simulink model "Referencegentest"  (R2023b)
settings: Solver=VariableStepAuto  StartTime=0.0  StopTime=2  RelTol=1e-3
libraries: spsCurrentMeasurementLib x7, spsSeriesRLCBranchLib x7, spsIGBTDiodeLib x4, spsVoltageMeasurementLib x4, eeGeneralControl x4, spsPLLLib x3, slpidlib x2, spsAlphaBetaZerotodq0Lib x2, spsabctoAlphaBetaZeroLib x2, spsACVoltageSourceLib x1, spsBreakerLib x1, spsDCVoltageSourceLib x1
settings Model: Creator=Jia Yee Wong  LastModifiedBy=Jia Yee Wong
settings SFSimCC: SimCustomHeaderCode="#include \"referencegen.h\""  SimUserSources=referencegen.cpp;  SimTargetLang=C++

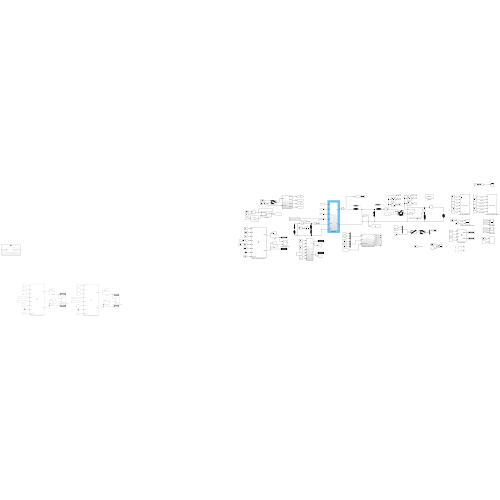
[thumbnail: Simulink's stored preview of the top-level diagram]
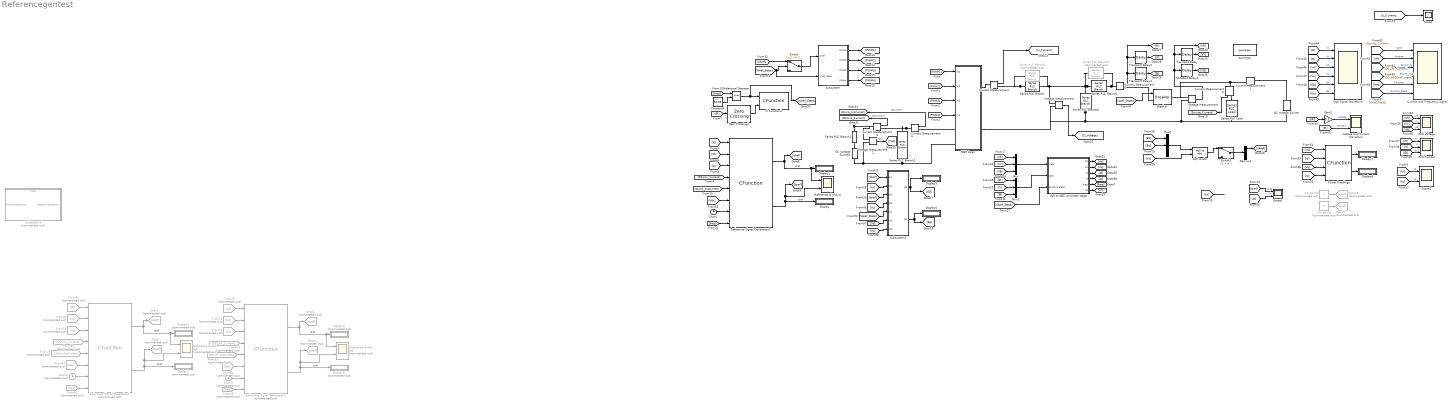
== system Referencegentest ==
  AC Voltage Source : spsACVoltageSourceLib/AC Voltage Source  Amplitude=340  Phase=0  Frequency=50  SampleTime=0  Measurements=None  BusType=PV  Pref=100  Qref=100  Qmin=-inf  Qmax=+inf
  Breaker : spsBreakerLib/Breaker  InitialState=0  SwitchingTimes="[1/60  5/60]"  External=on  BreakerResistance=0.00001  SnubberResistance=30  SnubberCapacitance=47e-9  Measurements=None  MoreParameters=on  NoBreakLoop=off
  C Function1 : CFunction  OutputCode=|  SampleTime=1/50000
      | if(Frequency == true && ZeroCross == 1){
      |     Output = 1;}
      | else if(Frequency == false){
      |         Output = 0;}
  Clock1 : Clock
  Clock2 : Clock  Commented=on
  Clock3 : Clock  Commented=on
  Constant4 : Constant  Value=50.05  SampleTime=1/50000
  Constant5 : Constant  Commented=on
  Constant6 : Constant  Commented=on  Value=0
  Current Measurement{,1..5} (6 alike) : spsCurrentMeasurementLib/Current Measurement  PhasorSimulation=off  OutputType=Complex  PSBequivalent=0
  Current and Frequency Signal : Scope  NumInputPorts=6
  DC Voltage Source1 : spsDCVoltageSourceLib/DC Voltage Source  Amplitude=400  Measurements=None
  Demux4 : Demux  Outputs=3
  Display{,1,4..7} (6 alike) : Display
  Display{2..3,8..9} (4 alike) : Display  Commented=on
  Dq0 Signal Waveform : Scope  NumInputPorts=6
  From26 : From  Commented=on  GotoTag=DCLink_OutCurrent
  From30 : From  Commented=on  GotoTag=Vdc
  From31 : From  Commented=on  GotoTag=freq
  From33 : From  Commented=on  GotoTag=DCLink_Current
  From41 : From  Commented=on  GotoTag=Id
  From42 : From  Commented=on  GotoTag=Vd
  From50 : From  Commented=on  GotoTag=Iq
  From51 : From  Commented=on  GotoTag=DCLink_OutCurrent
  From61 : From  Commented=on  GotoTag=Vdc
  From68 : From  Commented=on  GotoTag=freq
  From69 : From  Commented=on  GotoTag=DCLink_Current
  From70 : From  Commented=on  GotoTag=Id
  From71 : From  Commented=on  GotoTag=Vd
  From72 : From  Commented=on  GotoTag=Iq
  Gain2 : Gain  Gain=0.2
  Goto1 : Goto  Commented=on  GotoTag=Idref
  Goto2 : Goto  Commented=on  GotoTag=Iqref
  Goto3 : Goto  Commented=on  GotoTag=Idref
  Goto36 : Goto  Commented=on  GotoTag=Idref
  Goto37 : Goto  Commented=on  GotoTag=Iqref
  Goto4 : Goto  Commented=on  GotoTag=Iqref
  Grid Current : Scope  NumInputPorts=3
  Grid Voltage : Scope  NumInputPorts=3
  IGBT Array : Subsystem
  Mux : Mux  Inputs=3
  Mux1 : Mux  Inputs=3
  Mux2 : Mux  Inputs=3
  Power Readings : CFunction  OutputCode=|
      | PTotal = Id*Vd;
      | QTotal = Id*Vq-Vq*Id;
  Reference Id and Iq : Scope  NumInputPorts=2
  Reference Id and Iq1 : Scope  Commented=on  NumInputPorts=2
  Reference Id and Iq2 : Scope  Commented=on  NumInputPorts=2
  Reference Signal Generation1 : CFunction  Commented=on  OutputCode=|  StartCode=|  SampleTime=1/50000
      OutputCode=|
      | if(Id!=PreviousId || Iq!=PreviousIq){
      |     if(ReferenceGenTrigger(Freq_PLL)){
      |         Idref=IdrefCalc(CLK,Vd,Iin,Iout, Vdc, Vdc);
      |   //Idref =1;
      |    Iqref=0;
      |    PreviousId=Id;
      |    PreviousIq=Iq;
      |    }
      |   
      | } else { Idref = 0; Iqref = 0;}
      StartCode=|
      | PreviousIq =0;
      | PreviousId =0;
  Reference Signal Generation2 : CFunction  OutputCode=|  StartCode=|  SampleTime=1/50000
      OutputCode=|
      | if(Id!=PreviousId || Iq!=PreviousIq){
      |     if(ReferenceGenTrigger(Freq_PLL)){
      |        // Idref=IdrefCalc(CLK,Vd,Iin,Iout, Vdc, Vdc);
      |   Idref =1000/Vd;
      |    Iqref=0;
      |    PreviousId=Id;
      |    PreviousIq=Iq;
      |    }
      |   
      | } else { Idref = 0; Iqref = 0;}
      StartCode=|
      | PreviousIq =0;
      | PreviousId =0;
  Reference Signal Generation3 : CFunction  Commented=on  OutputCode=|  StartCode=|  SampleTime=1/50000
      OutputCode=|
      | if(Id!=PreviousId || Iq!=PreviousIq){
      |     if(ReferenceGenTrigger(Freq_PLL)){
      |         Idref=IdrefCalc(CLK,Vd,Iin,Iout, Vdc, Vdc);
      |   //Idref =1;
      |    Iqref=0;
      |    PreviousId=Id;
      |    PreviousIq=Iq;
      |    }
      |   
      | } else { Idref = 0; Iqref = 0;}
      StartCode=|
      | PreviousIq =0;
      | PreviousId =0;
  Relational Operator : RelationalOperator  Operator=<=  OutDataTypeStr=boolean  RndMeth=Simplest  InputSameDT=off
  Scope : Scope
  Scope1 : Scope  NumInputPorts=2
  Scope2 : Scope  NumInputPorts=2
  Series RLC Branch : spsSeriesRLCBranchLib/Series RLC Branch  LConnTagsString=__new0  RConnTagsString=__new0  BranchType=L  Resistance=1  Inductance=20.4e-3  SetiL0=off  InitialCurrent=0  Capacitance=1e-6  Setx0=off  InitialVoltage=0  Measurements=None
  Series RLC Branch1 : spsSeriesRLCBranchLib/Series RLC Branch  LConnTagsString=__new0  RConnTagsString=__new0  BranchType=L  Resistance=1  Inductance=148.336e-6  SetiL0=off  InitialCurrent=0  Capacitance=1e-6  Setx0=off  InitialVoltage=0  Measurements=None
  Series RLC Branch2 : spsSeriesRLCBranchLib/Series RLC Branch  LConnTagsString=__new0  RConnTagsString=__new0  BranchType=RC  Resistance=1  Inductance=0  SetiL0=off  InitialCurrent=0  Capacitance=47e-3  Setx0=off  InitialVoltage=300  Measurements=None
  Series RLC Branch3 : spsSeriesRLCBranchLib/Series RLC Branch  LConnTagsString=__new0  RConnTagsString=__new0  BranchType=RL  Resistance=10  Inductance=0  SetiL0=off  InitialCurrent=0  Capacitance=1e-6  Setx0=off  InitialVoltage=0  Measurements=None
  Series RLC Branch4 : spsSeriesRLCBranchLib/Series RLC Branch  Commented=on  LConnTagsString=__new0  RConnTagsString=__new0  BranchType=R  Resistance=220  Inductance=20.4e-3  SetiL0=off  InitialCurrent=0  Capacitance=1e-6  Setx0=off  InitialVoltage=0  Measurements=None
  Series RLC Branch5 : spsSeriesRLCBranchLib/Series RLC Branch  Commented=on  LConnTagsString=__new0  RConnTagsString=__new0  BranchType=R  Resistance=220  Inductance=20.4e-3  SetiL0=off  InitialCurrent=0  Capacitance=1e-6  Setx0=off  InitialVoltage=0  Measurements=None
  Series RLC Branch8 : spsSeriesRLCBranchLib/Series RLC Branch  LConnTagsString=__new0  RConnTagsString=__new0  BranchType=RC  Resistance=120  Inductance=100e-6  SetiL0=off  InitialCurrent=0  Capacitance=5.526e-6  Setx0=off  InitialVoltage=0  Measurements=None
  Series RLC Load : spsSeriesRLCLoadLib/Series RLC Load  LConnTagsString=a  RConnTagsString=__new0  NominalVoltage=240  NominalFrequency=50  ActivePower=10e2  InductivePower=0  CapacitivePower=0  Setx0=off  InitialVoltage=240  SetiL0=off  InitialCurrent=10  Measurements=None  LoadType=constant PQ
  Subsystem : Subsystem
  Subsystem3 : Subsystem
  Subsystem5 : Subsystem  Commented=on
  Switch : Switch  Threshold=1  SaturateOnIntegerOverflow=off  InputSameDT=off
  Switch5 : Switch  Threshold=1  SaturateOnIntegerOverflow=off  InputSameDT=off
  Transport Delay : TransportDelay  DelayTime=6.67e-3  BufferSize=4096
  Transport Delay1 : TransportDelay  DelayTime=13.34e-3  BufferSize=5120
  Transport Delay2 : TransportDelay  DelayTime=6.67e-3  BufferSize=4096
  Transport Delay3 : TransportDelay  DelayTime=13.34e-3  BufferSize=4096
  Voltage Measurement : spsVoltageMeasurementLib/Voltage Measurement  PhasorSimulation=off  OutputType=Complex  PSBequivalent=0
  Voltage Measurement1 : spsVoltageMeasurementLib/Voltage Measurement  PhasorSimulation=off  OutputType=Complex  PSBequivalent=0
  Voltage Measurement2 : spsVoltageMeasurementLib/Voltage Measurement  PhasorSimulation=off  OutputType=Complex  PSBequivalent=0
  Voltage and Current Waveform : Scope  NumInputPorts=2
  Zero Crossing1 : dspsigops/Zero Crossing
  dq0 to ABC converter stage : Subsystem
  dq0 to abc : spsdq0toabcLib/dq0 to abc  Alignment=90 degrees behind phase A axis
  powergui : spspowerguiLib/powergui  Priority=1  SimulationMode=Continuous  SampleTime=50e-6  frequency=60  Iterations=50  frequencyindice=0  Pbase=100e6  ErrMax=1e-4  UnitsV=kV  UnitsW=MW  buscounter=0  FunctionMessages=off  echomessages=off  EnableUseOfTLC=off  CurrentSourceSwitches=off  DisableSnubberDevices=off  DisableRonSwitches=off  DisableVfSwitches=off  DisplayEquations=off  AutomaticDiscreteSolvers=off  SolverType=Tustin/Backward Euler (TBE)  Interpol=off  ExternalGateDelay=off  methode=off  Ts=100  x0status=blocks  SPID=on  SwTol=0  HookPort=off  NonlinearTolerance=1e-4  nMaxIteration=100  ContinueOnMaxIteration=off  RestoreLinks=warning  ResistiveCurrentMeasurement=off  Frange=[0:2:500]  Ylog=off  Xlog=on  ShowGrid=off  save=off  variable=ZData  structure=0  ZoomFFT=off  StartTime=0.0  cycles=1  DisplayStyle=1  fundamental=60  FreqAxis=off  MaxFrequency=1000  frequencyindicesteady=1  RmsSteady=1  display=off
  wires:
  [IR] -> Voltage and Current Waveform/2  "Current"
  Clock1/1 -> Reference Signal Generation2/7
  [Vq] -> Subsystem3/7(In6)
  [Iq] -> Power Readings/4
  Subsystem/4(PWM4) -> [PWM4]
  [VAref_State] -> dq0 to ABC converter stage/3(Synchro State)
  [VAref_State] -> Subsystem3/5(In2)
  Switch/1 -> Subsystem/1(Vref)
  Constant5/1 -> Goto36/1
  [Iq] -> Subsystem3/4(In8)
  [Vdc] -> Reference Signal Generation2/6
  [Id] -> Power Readings/2
  [DCLink_Current] -> Reference Signal Generation2/4
  Reference Signal Generation2/2 -> Reference Id and Iq/2, [Iqref], Display/1  "Iqref"
  [IR] -> Mux1/1
  dq0 to ABC converter stage/2(Vq) -> [Vq]
  [Iq] -> Reference Signal Generation2/3
  [Id] -> Subsystem3/2(In4)
  Current Measurement3/1 -> [DCLink_Current]  "DCLinkOut"
  Transport Delay3/1 -> [IB]
  dq0 to ABC converter stage/4(Iq) -> [Iq]
  Switch5/1 -> Demux4/1
  Mux/1 -> dq0 to ABC converter stage/1(Vabc)
  Subsystem3/1(Ed) -> [ED], Display5/1
  [VY] -> Grid Voltage/2  "VY"
  [VR] -> Mux/1
  [IY] -> Grid Current/2  "IY"
  dq0 to abc/1 -> Switch5/1
  Subsystem/1(PWM1) -> [PWM1]
  [VR] -> Grid Voltage/1  "VR"
  [wt] -> dq0 to abc/2
  [VAref] -> Switch/1
  [freq] -> Relational Operator/1
  Constant4/1 -> Relational Operator/2
  [VB] -> Grid Voltage/3  "VB"
  Subsystem/2(PWM2) -> [PWM2]
  Current Measurement/1 -> [Li_Current]
  Transport Delay1/1 -> [VB]
  Transport Delay2/1 -> [IY]
  Transport Delay/1 -> [VY]
  Mux2/1 -> dq0 to abc/1
  dq0 to ABC converter stage/3(Id) -> [Id]
  [VAref_State] -> Breaker/1
  [VR] -> Gain2/1
  Relational Operator/1 -> [VAref_State], C Function1/1
  [freq] -> Reference Signal Generation2/8
  dq0 to ABC converter stage/5(freq) -> [freq]
  [Eq] -> Mux2/2
  [IR] -> Current and Frequency Signal/2  "Iinverter"
  [Id] -> Scope2/1  "Id"
  Constant6/1 -> Goto37/1
  [Vd] -> Dq0 Signal Waveform/3  "Vd"
  Zero Crossing1/1 -> C Function1/2
  Current Measurement4/1 -> [DCLink_OutCurrent]  "DCLinkIN"
  [IR] -> Zero Crossing1/1
  [Source_Current] -> Current and Frequency Signal/1  "Igrid"
  [VAref_State] -> Current and Frequency Signal/6  "Synchro_State"
  Voltage Measurement2/1 -> [Vdc]  "VDC"
  [Iqref] -> Subsystem3/3(In5)
  Current Measurement1/1 -> [IR], Transport Delay2/1, Transport Delay3/1
  Gain2/1 -> Voltage and Current Waveform/1  "Voltage"
  [Vq] -> Dq0 Signal Waveform/4  "Vq"
  Subsystem/3(PWM3) -> [PWM3]
  [IB] -> Grid Current/3  "IB"
  [Vd] -> Reference Signal Generation2/2
  [DCLink_OutCurrent] -> Current and Frequency Signal/4  "DCLink_Out"
  [Id] -> Reference Signal Generation2/1
  [PWM2] -> IGBT Array/2(In1)
  [DCLink_Current] -> Current and Frequency Signal/3  "DcLink_IN"
  dq0 to ABC converter stage/1(Vd) -> [Vd]
  [ED] -> Mux2/1
  [PWM3] -> IGBT Array/3(In3)
  [ED] -> Dq0 Signal Waveform/5  "Ed"
  Voltage Measurement1/1 -> [VR], Transport Delay/1, Transport Delay1/1
  [IY] -> Mux1/2
  [Idref] -> Subsystem3/1(In1)
  [VY] -> Mux/2
  Power Readings/1 -> Display7/1
  [IR] -> Grid Current/1  "IR"
  [Vq] -> Power Readings/3
  [PWM1] -> IGBT Array/1(In2)
  [IB] -> Mux1/3
  [VB] -> Mux/3
  [Vd] -> Power Readings/1
  Power Readings/2 -> Display4/1
  Reference Signal Generation2/1 -> Reference Id and Iq/1, Display1/1, [Idref]  "Idref"
  [PWM4] -> IGBT Array/4(In4)
  Demux4/1 -> [VAref]
  Voltage Measurement/1 -> [Ci_Voltage]
  Current Measurement5/1 -> [Source_Current]
  Subsystem3/2(Eq) -> [Eq], Display6/1
  dq0 to ABC converter stage/6(wt) -> [wt]
  [DCLink_OutCurrent] -> Reference Signal Generation2/5
  [freq] -> Current and Frequency Signal/5  "FSystem"
  Mux1/1 -> dq0 to ABC converter stage/2(IAbc)
  [Id] -> Dq0 Signal Waveform/1  "Id"
  [Iq] -> Dq0 Signal Waveform/2  "Iq"
  [Eq] -> Dq0 Signal Waveform/6  "Eq"
  [Iq] -> Scope2/2  "Iq"
  [Vd] -> Subsystem3/6(In3)
  [VAref_State] -> Subsystem/2(Vref_state), Switch/2
  Reference Signal Generation1/1 -> Reference Id and Iq1/1, Display3/1, Goto1/1  "Idref"
  From26/1 -> Reference Signal Generation1/5
  From42/1 -> Reference Signal Generation1/2
  From50/1 -> Reference Signal Generation1/3
  From31/1 -> Reference Signal Generation1/8
  Reference Signal Generation1/2 -> Reference Id and Iq1/2, Goto2/1, Display2/1  "Iqref"
  Clock2/1 -> Reference Signal Generation1/7
  From30/1 -> Reference Signal Generation1/6
  From33/1 -> Reference Signal Generation1/4
  From41/1 -> Reference Signal Generation1/1
  From70/1 -> Reference Signal Generation3/1
  Clock3/1 -> Reference Signal Generation3/7
  From69/1 -> Reference Signal Generation3/4
  Reference Signal Generation3/2 -> Reference Id and Iq2/2, Goto4/1, Display8/1  "Iqref"
  From68/1 -> Reference Signal Generation3/8
  From61/1 -> Reference Signal Generation3/6
  From72/1 -> Reference Signal Generation3/3
  From71/1 -> Reference Signal Generation3/2
  From51/1 -> Reference Signal Generation3/5
  Reference Signal Generation3/1 -> Reference Id and Iq2/1, Display9/1, Goto3/1  "Idref"
  [Id] -> Scope1/2  "Id"
  [Idref] -> Scope1/1  "Idref"
  [Li_Current] -> Scope/1
  [wt] -> ?
  connections:
  Current Measurement4/LConn1 -- Current Measurement3/RConn1 -- Series RLC Branch2/LConn1
  Series RLC Branch8/RConn1 -- IGBT Array/RConn2 -- Voltage Measurement/LConn2 -- AC Voltage Source/LConn1 -- Series RLC Load/RConn1 -- Voltage Measurement1/LConn2
  Voltage Measurement2/LConn2 -- Series RLC Branch2/RConn1 -- IGBT Array/LConn2 -- DC Voltage Source1/LConn1
  Series RLC Branch1/LConn1 -- Series RLC Branch8/LConn1 -- Series RLC Branch5/LConn1 -- Voltage Measurement/LConn1 -- Series RLC Branch/RConn1 -- Series RLC Branch4/RConn1
  Series RLC Branch3/LConn1 -- Current Measurement3/LConn1 -- Voltage Measurement2/LConn1
  Current Measurement1/LConn1 -- Series RLC Branch5/RConn1 -- Series RLC Branch1/RConn1
  Current Measurement2/RConn1 -- Breaker/RConn1 -- Voltage Measurement1/LConn1 -- Current Measurement5/LConn1
  Series RLC Branch/LConn1 -- Current Measurement/RConn1 -- Series RLC Branch4/LConn1
  IGBT Array/RConn1 -- Current Measurement/LConn1
  Current Measurement4/RConn1 -- IGBT Array/LConn1
  Breaker/LConn1 -- Current Measurement1/RConn1
  Current Measurement2/LConn1 -- AC Voltage Source/RConn1
  Current Measurement5/RConn1 -- Series RLC Load/LConn1
  Series RLC Branch3/RConn1 -- DC Voltage Source1/RConn1

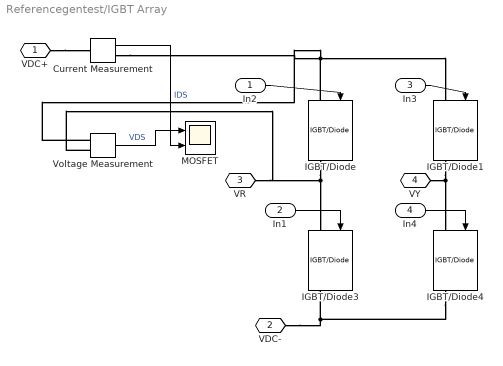
== system Referencegentest/IGBT Array ==
  In2 : Inport
  In1 : Inport  Port=2
  In3 : Inport  Port=3
  In4 : Inport  Port=4
  Current Measurement : spsCurrentMeasurementLib/Current Measurement  PhasorSimulation=off  OutputType=Complex  PSBequivalent=0
  IGBT/Diode{,1,3..4} (4 alike) : spsIGBTDiodeLib/IGBT//Diode  Ron=1e-3  Rs=1e5  Cs=inf  Measurements=on
  MOSFET : Scope  NumInputPorts=2
  Voltage Measurement : spsVoltageMeasurementLib/Voltage Measurement  PhasorSimulation=off  OutputType=Complex  PSBequivalent=0
  VDC+ : PMIOPort  Side=Left
  VDC- : PMIOPort  Port=2  Side=Left
  VR : PMIOPort  Port=3  Side=Right
  VY : PMIOPort  Port=4  Side=Right
  wires:
  In1/1 -> IGBT/Diode3/1
  In4/1 -> IGBT/Diode4/1
  In3/1 -> IGBT/Diode1/1
  In2/1 -> IGBT/Diode/1
  Voltage Measurement/1 -> MOSFET/1  "VDS"
  Current Measurement/1 -> MOSFET/2  "IDS"
  connections:
  IGBT/Diode4/RConn1 -- VDC-/RConn1 -- IGBT/Diode3/RConn1
  IGBT/Diode/RConn1 -- Voltage Measurement/LConn2 -- VR/RConn1 -- IGBT/Diode3/LConn1
  IGBT/Diode1/RConn1 -- VY/RConn1 -- IGBT/Diode4/LConn1
  IGBT/Diode/LConn1 -- Current Measurement/RConn1 -- Voltage Measurement/LConn1 -- IGBT/Diode1/LConn1
  VDC+/RConn1 -- Current Measurement/LConn1

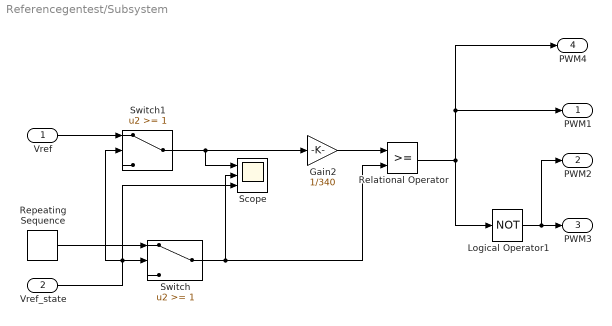
== system Referencegentest/Subsystem ==
  Vref : Inport
  Vref_state : Inport  Port=2
  Gain2 : Gain  Gain=1/340
  Logical Operator1 : Logic  Operator=NOT  AllPortsSameDT=off  OutDataTypeStr=boolean
  Relational Operator : RelationalOperator  OutDataTypeStr=boolean  RndMeth=Simplest  InputSameDT=off
  Repeating Sequence : simulink/Sources/Repeating Sequence  rep_seq_t=[0 0.00005 0.0001]  rep_seq_y=[-1 1 -1]
  Scope : Scope  NumInputPorts=3
  Switch : Switch  Threshold=1  SaturateOnIntegerOverflow=off  InputSameDT=off
  Switch1 : Switch  Threshold=1  SaturateOnIntegerOverflow=off  InputSameDT=off
  PWM1 : Outport
  PWM2 : Outport  Port=2
  PWM3 : Outport  Port=3
  PWM4 : Outport  Port=4
  wires:
  Gain2/1 -> Relational Operator/1
  Relational Operator/1 -> Logical Operator1/1, PWM1/1, PWM4/1
  Logical Operator1/1 -> PWM2/1, PWM3/1
  Repeating Sequence/1 -> Switch/1
  Switch/1 -> Scope/2, Relational Operator/2
  Vref_state/1 -> Scope/3, Switch1/2, Switch/2
  Switch1/1 -> Gain2/1, Scope/1
  Vref/1 -> Switch1/1

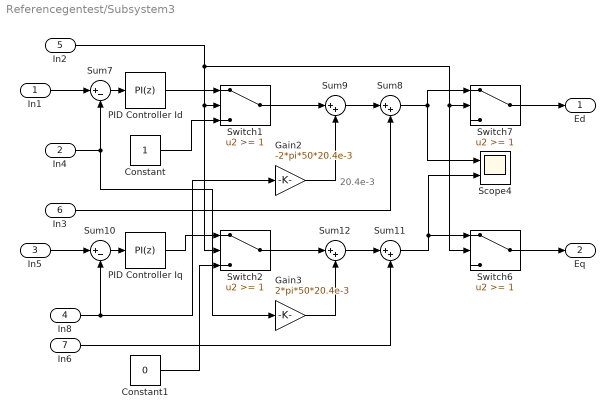
== system Referencegentest/Subsystem3 ==
  note: 20.4e-3
  In1 : Inport
  In4 : Inport  Port=2
  In5 : Inport  Port=3
  In8 : Inport  Port=4
  In2 : Inport  Port=5
  In3 : Inport  Port=6
  In6 : Inport  Port=7
  Constant : Constant
  Constant1 : Constant  Value=0
  Gain2 : Gain  Gain=-2*pi*50*20.4e-3
  Gain3 : Gain  Gain=2*pi*50*20.4e-3
  PID Controller Id : slpidlib/PID Controller  Controller=PI  Form=Parallel  TimeDomain=Discrete-time  UseExternalTs=off  SampleTime=5e-5  IntegratorMethod=Forward Euler  FilterMethod=Forward Euler  ControllerParametersSource=internal  P=500  I=100  UseKiTs=on  D=0.2  N=100  UseFilter=on  TunerSelectOption=Transfer Function Based (PID Tuner App)  InitialConditionSource=internal  InitialConditionForIntegrator=0  InitialConditionForFilter=0  DifferentiatorICPrevScaledInput=0  ExternalReset=none  TrackingMode=off  Kt=1  LimitOutput=on  SatLimitsSource=internal  UpperSaturationLimit=200  LowerSaturationLimit=-200  LinearizeAsGain=on  AntiWindupMode=back-calculation  Kb=1  LimitIntegrator=off  UpperIntegratorSaturationLimit=inf  LowerIntegratorSaturationLimit=-inf  POutMin=[]  POutMax=[]  IOutMin=[]  IOutMax=[]  DOutMin=[]  DOutMax=[]  NOutMin=[]  NOutMax=[]  SumOutMin=[]  SumOutMax=[]  SaturationOutMin=[]  SaturationOutMax=[]  PParamMin=[]  PParamMax=[]  IParamMin=[]  IParamMax=[]  DParamMin=[]  DParamMax=[]  NParamMin=[]  NParamMax=[]  KbParamMin=[]  KbParamMax=[]  KtParamMin=[]  KtParamMax=[]  KbOutMin=[]  KbOutMax=[]  KtOutMin=[]  KtOutMax=[]  IntegratorOutMin=[]  IntegratorOutMax=[]  FilterOutMin=[]  FilterOutMax=[]  SumI1OutMin=[]  SumI1OutMax=[]  SumI2OutMin=[]  SumI2OutMax=[]  SumI3OutMin=[]  SumI3OutMax=[]  SumI4OutMin=[]  SumI4OutMax=[]  SumDOutMin=[]  SumDOutMax=[]  DifferentiatorOutMin=[]  DifferentiatorOutMax=[]  FilterDiffOutCoefMin=[]  FilterDiffOutCoefMax=[]  ReciprocalOutMin=[]  ReciprocalOutMax=[]  SumDenOutMin=[]  SumDenOutMax=[]  SumNumOutMin=[]  SumNumOutMax=[]  DivideOutMin=[]  DivideOutMax=[]  UdiffTsProdOutMin=[]  UdiffTsProdOutMax=[]  NTsProdOutMin=[]  NTsProdOutMax=[]  UintegralTsProdOutMin=[]  UintegralTsProdOutMax=[]  UngainTsProdOutMin=[]  UngainTsProdOutMax=[]  ClampingZeroOutDataTypeStr=Inherit: Inherit via back propagation  ClampingZeroOutMin=[]  ClampingZeroOutMax=[]  FilterDenConstantOutDataTypeStr=Inherit: Inherit via back propagation  FilterDenConstantOutMin=[]  FilterDenConstantOutMax=[]  PCopyOutDataTypeStr=Inherit: Inherit via back propagation  PCopyOutMin=[]  PCopyOutMax=[]  NCopyOutDataTypeStr=Inherit: Inherit via back propagation  NCopyOutMin=[]  NCopyOutMax=[]  IntegratorContinuousStateAttributes=''  IntegratorStateIdentifier=Id  IntegratorStateMustResolveToSignalObject=off  IntegratorRTWStateStorageClass=Auto  FilterContinuousStateAttributes=''  FilterStateMustResolveToSignalObject=off  FilterRTWStateStorageClass=Auto  ParallelPVariant=InternalParameters  IdealPVariant=Disabled  IVariant=InternalParameters  DVariant=Disabled  IntegratorVariant=Discrete  SatVariant=Enabled  AWVariant=BackCalculation  PCopyVariant=Disabled  TRVariant=Disabled  FdbkBlocksVariant=Forward  IdealPFdbkVariant=Disabled  SatFdbkVariant=Disabled  DerivativeFilterVariant=Disabled  NVariant=Disabled  NCopyVariant=Disabled_SignalSpec  FilterICVariant=Disabled  IntegratorICVariant=InternalICs  ExternalResetVariant=Disabled  TRSumVariant=Passthrough  SumFdbkVariant=Disabled  SumVariant=Sum_PI  TsampFilterVariant=InternalTs  TsampNgainVariant=Passthrough  TsampIntegralVariant=Disabled_SignalSpec  ExternalSaturationOutDataTypeStr=Inherit: Same as second input
  PID Controller Iq : slpidlib/PID Controller  Controller=PI  Form=Parallel  TimeDomain=Discrete-time  UseExternalTs=off  SampleTime=5e-5  IntegratorMethod=Forward Euler  FilterMethod=Forward Euler  ControllerParametersSource=internal  P=500  I=100  UseKiTs=on  D=0.2  N=100  UseFilter=on  TunerSelectOption=Transfer Function Based (PID Tuner App)  InitialConditionSource=internal  InitialConditionForIntegrator=0  InitialConditionForFilter=0  DifferentiatorICPrevScaledInput=0  ExternalReset=none  TrackingMode=off  Kt=1  LimitOutput=on  SatLimitsSource=internal  UpperSaturationLimit=200  LowerSaturationLimit=-200  LinearizeAsGain=on  AntiWindupMode=back-calculation  Kb=1  LimitIntegrator=off  UpperIntegratorSaturationLimit=inf  LowerIntegratorSaturationLimit=-inf  POutMin=[]  POutMax=[]  IOutMin=[]  IOutMax=[]  DOutMin=[]  DOutMax=[]  NOutMin=[]  NOutMax=[]  SumOutMin=[]  SumOutMax=[]  SaturationOutMin=[]  SaturationOutMax=[]  PParamMin=[]  PParamMax=[]  IParamMin=[]  IParamMax=[]  DParamMin=[]  DParamMax=[]  NParamMin=[]  NParamMax=[]  KbParamMin=[]  KbParamMax=[]  KtParamMin=[]  KtParamMax=[]  KbOutMin=[]  KbOutMax=[]  KtOutMin=[]  KtOutMax=[]  IntegratorOutMin=[]  IntegratorOutMax=[]  FilterOutMin=[]  FilterOutMax=[]  SumI1OutMin=[]  SumI1OutMax=[]  SumI2OutMin=[]  SumI2OutMax=[]  SumI3OutMin=[]  SumI3OutMax=[]  SumI4OutMin=[]  SumI4OutMax=[]  SumDOutMin=[]  SumDOutMax=[]  DifferentiatorOutMin=[]  DifferentiatorOutMax=[]  FilterDiffOutCoefMin=[]  FilterDiffOutCoefMax=[]  ReciprocalOutMin=[]  ReciprocalOutMax=[]  SumDenOutMin=[]  SumDenOutMax=[]  SumNumOutMin=[]  SumNumOutMax=[]  DivideOutMin=[]  DivideOutMax=[]  UdiffTsProdOutMin=[]  UdiffTsProdOutMax=[]  NTsProdOutMin=[]  NTsProdOutMax=[]  UintegralTsProdOutMin=[]  UintegralTsProdOutMax=[]  UngainTsProdOutMin=[]  UngainTsProdOutMax=[]  ClampingZeroOutDataTypeStr=Inherit: Inherit via back propagation  ClampingZeroOutMin=[]  ClampingZeroOutMax=[]  FilterDenConstantOutDataTypeStr=Inherit: Inherit via back propagation  FilterDenConstantOutMin=[]  FilterDenConstantOutMax=[]  PCopyOutDataTypeStr=Inherit: Inherit via back propagation  PCopyOutMin=[]  PCopyOutMax=[]  NCopyOutDataTypeStr=Inherit: Inherit via back propagation  NCopyOutMin=[]  NCopyOutMax=[]  IntegratorContinuousStateAttributes=''  IntegratorStateIdentifier=Id  IntegratorStateMustResolveToSignalObject=off  IntegratorRTWStateStorageClass=Auto  FilterContinuousStateAttributes=''  FilterStateMustResolveToSignalObject=off  FilterRTWStateStorageClass=Auto  ParallelPVariant=InternalParameters  IdealPVariant=Disabled  IVariant=InternalParameters  DVariant=Disabled  IntegratorVariant=Discrete  SatVariant=Enabled  AWVariant=BackCalculation  PCopyVariant=Disabled  TRVariant=Disabled  FdbkBlocksVariant=Forward  IdealPFdbkVariant=Disabled  SatFdbkVariant=Disabled  DerivativeFilterVariant=Disabled  NVariant=Disabled  NCopyVariant=Disabled_SignalSpec  FilterICVariant=Disabled  IntegratorICVariant=InternalICs  ExternalResetVariant=Disabled  TRSumVariant=Passthrough  SumFdbkVariant=Disabled  SumVariant=Sum_PI  TsampFilterVariant=InternalTs  TsampNgainVariant=Passthrough  TsampIntegralVariant=Disabled_SignalSpec  ExternalSaturationOutDataTypeStr=Inherit: Same as second input
  Scope4 : Scope  NumInputPorts=2
  Sum10 : Sum  Inputs=|+-
  Sum{8..9,11..12} (4 alike) : Sum  Inputs=|++
  Sum7 : Sum  Inputs=|+-
  Switch{1..2,6..7} (4 alike) : Switch  Threshold=1  SaturateOnIntegerOverflow=off  InputSameDT=off
  Ed : Outport
  Eq : Outport  Port=2
  wires:
  Switch1/1 -> Sum9/1
  In5/1 -> Sum10/1
  In1/1 -> Sum7/1
  In6/1 -> Sum11/2
  In2/1 -> Switch6/2, Switch7/2, Switch2/2, Switch1/2
  Switch7/1 -> Ed/1
  Sum8/1 -> Scope4/1, Switch7/1
  Sum10/1 -> PID Controller Iq/1
  Sum11/1 -> Switch6/1, Scope4/2
  Gain3/1 -> Sum12/2
  Sum7/1 -> PID Controller Id/1
  PID Controller Iq/1 -> Switch2/1
  In3/1 -> Sum8/2
  Sum9/1 -> Sum8/1
  Gain2/1 -> Sum9/2
  Sum12/1 -> Sum11/1
  In4/1 -> Gain3/1, Sum7/2
  In8/1 -> Gain2/1, Sum10/2
  PID Controller Id/1 -> Switch1/1
  Switch2/1 -> Sum12/1
  Switch6/1 -> Eq/1
  Constant/1 -> Switch1/3
  Constant1/1 -> Switch2/3

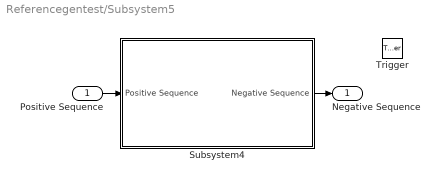
== system Referencegentest/Subsystem5 ==
  Positive Sequence : Inport
  Trigger : TriggerPort  VariantControl=(inherit)  PortDimensions=1
  Subsystem4 : Subsystem
  Negative Sequence : Outport
  wires:
  Subsystem4/1(Negative Sequence) -> Negative Sequence/1
  Positive Sequence/1 -> Subsystem4/1(Positive Sequence)

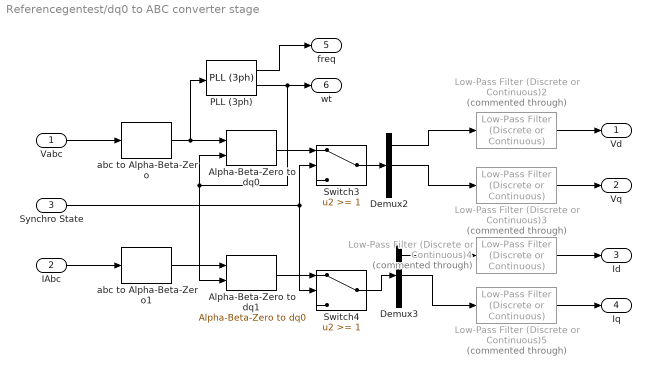
== system Referencegentest/dq0 to ABC converter stage ==
  Vabc : Inport
  IAbc : Inport  Port=2
  Synchro State : Inport  Port=3
  Alpha-Beta-Zero to dq0 : spsAlphaBetaZerotodq0Lib/Alpha-Beta-Zero to dq0  Alignment=90 degrees behind phase A axis
  Alpha-Beta-Zero to dq1 : spsAlphaBetaZerotodq0Lib/Alpha-Beta-Zero to dq0  Alignment=90 degrees behind phase A axis
  Demux2 : Demux  Outputs=3
  Demux3 : Demux  Outputs=3
  Low-Pass Filter (Discrete or Continuous){2..5} (4 alike) : eeGeneralControl/Low-Pass Filter (Discrete or Continuous)  Commented=through  K=1  T=2*pi*50  B=inf  A=-inf  init_option=Inherited from block input  x0=0  Ts=0
  PLL (3ph) : spsPLL3phLib/PLL (3ph)  Fmin=45  Par_Init=[0, 60]  ParK=[180, 3200, 1]  TcD=1e-4  MaxRateChangeFreq=12  FilterCutOffFreq=25  Ts=0  AGC=on
  Switch3 : Switch  Threshold=1  SaturateOnIntegerOverflow=off  InputSameDT=off
  Switch4 : Switch  Threshold=1  SaturateOnIntegerOverflow=off  InputSameDT=off
  abc to Alpha-Beta-Zero : spsabctoAlphaBetaZeroLib/abc to Alpha-Beta-Zero
  abc to Alpha-Beta-Zero1 : spsabctoAlphaBetaZeroLib/abc to Alpha-Beta-Zero
  Vd : Outport
  Vq : Outport  Port=2
  Id : Outport  Port=3
  Iq : Outport  Port=4
  freq : Outport  Port=5
  wt : Outport  Port=6
  wires:
  Demux3/2 -> Low-Pass Filter (Discrete or Continuous)5/1
  Synchro State/1 -> Switch4/2, Switch3/2
  Demux3/1 -> Low-Pass Filter (Discrete or Continuous)4/1
  Low-Pass Filter (Discrete or Continuous)5/1 -> Iq/1
  abc to Alpha-Beta-Zero1/1 -> Alpha-Beta-Zero to dq1/1
  Low-Pass Filter (Discrete or Continuous)4/1 -> Id/1
  Switch4/1 -> Demux3/1
  Demux2/2 -> Low-Pass Filter (Discrete or Continuous)3/1
  Low-Pass Filter (Discrete or Continuous)2/1 -> Vd/1
  Alpha-Beta-Zero to dq1/1 -> Switch4/1
  Demux2/1 -> Low-Pass Filter (Discrete or Continuous)2/1
  Low-Pass Filter (Discrete or Continuous)3/1 -> Vq/1
  Switch3/1 -> Demux2/1
  PLL (3ph)/1 -> freq/1
  Alpha-Beta-Zero to dq0/1 -> Switch3/1
  abc to Alpha-Beta-Zero/1 -> PLL (3ph)/1, Alpha-Beta-Zero to dq0/1
  Vabc/1 -> abc to Alpha-Beta-Zero/1
  PLL (3ph)/2 -> Alpha-Beta-Zero to dq1/2, Alpha-Beta-Zero to dq0/2, wt/1
  IAbc/1 -> abc to Alpha-Beta-Zero1/1

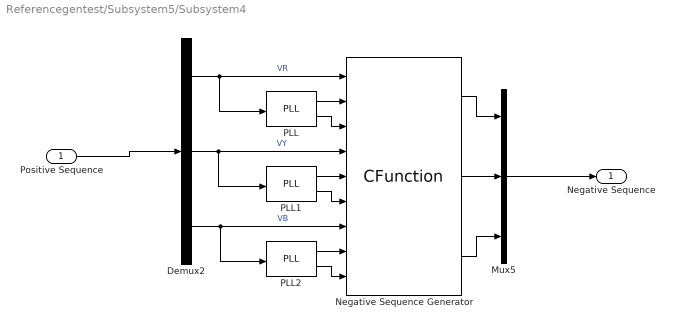
== system Referencegentest/Subsystem5/Subsystem4 ==
  Positive Sequence : Inport
  Demux2 : Demux  Outputs=3
  Mux5 : Mux  Inputs=3
  Negative Sequence Generator : CFunction  OutputCode=VaNeg = (NegativeSequenceVa(Va, Vb, Vc));
  PLL : spsPLLLib/PLL  Fmin=45  Par_Init=[0, 60]  ParK=[180, 3200, 1]  TcD=1e-4  MaxRateChangeFreq=12  FilterCutOffFreq=25  Ts=0  AGC=on
      settings: LibrarySourceBlock=sps_lib/Control/PLL
  PLL1 : spsPLLLib/PLL  Fmin=45  Par_Init=[0, 60]  ParK=[180, 3200, 1]  TcD=1e-4  MaxRateChangeFreq=12  FilterCutOffFreq=25  Ts=0  AGC=on
      settings: LibrarySourceBlock=sps_lib/Control/PLL
  PLL2 : spsPLLLib/PLL  Fmin=45  Par_Init=[0, 60]  ParK=[180, 3200, 1]  TcD=1e-4  MaxRateChangeFreq=12  FilterCutOffFreq=25  Ts=0  AGC=on
      settings: LibrarySourceBlock=sps_lib/Control/PLL
  Negative Sequence : Outport
  wires:
  Demux2/2 -> PLL1/1, Negative Sequence Generator/4  "VY"
  Positive Sequence/1 -> Demux2/1
  Demux2/3 -> PLL2/1, Negative Sequence Generator/7  "VB"
  Negative Sequence Generator/2 -> Mux5/2
  Demux2/1 -> PLL/1, Negative Sequence Generator/1  "VR"
  Mux5/1 -> Negative Sequence/1
  Negative Sequence Generator/1 -> Mux5/1
  Negative Sequence Generator/3 -> Mux5/3
  PLL/2 -> Negative Sequence Generator/3
  PLL2/1 -> Negative Sequence Generator/8
  PLL1/2 -> Negative Sequence Generator/6
  PLL/1 -> Negative Sequence Generator/2
  PLL2/2 -> Negative Sequence Generator/9
  PLL1/1 -> Negative Sequence Generator/5
